simulink model "TEST_Datcom"  (R2020b)
settings: Solver=FixedStepAuto  StartTime=0.0  StopTime=100  FixedStep=DATCOM_DYN.Ts  RelTol=1e-3
undefined symbols (not defined in the file or in its folder): DATCOM_DYN, Earth, F, Light, MIL, statdyn, WGS84
libraries: aerolibadyn x3, aerolibwind2 x3, aerolibasang x3, aerolibactuator x3, shared6dof x2, aerolibatmos2 x2, aerolibconvert2 x2, pid_lib x1, simulink_extras x1, aerolibtransform2 x1
settings Model: Creator=sl  LastModifiedBy=sl
settings OptimizationCC: DefaultParameterBehavior=Inlined  EnhancedBackFolding=on  PassReuseOutputArgsAs=Individual arguments  ZeroExternalMemoryAtStartup=off  ZeroInternalMemoryAtStartup=off  OptimizeBlockOrder=speed  DifferentSizesBufferReuse=on  OptimizationCustomize=off  EfficientTunableParamExpr=on
settings DebuggingCC: ParameterTunabilityLossMsg=error
settings HardwareCC: ProdBitPerPointer=32  ProdBitPerSizeT=32  ProdBitPerPtrDiffT=32  ProdLargestAtomicInteger=Long  ProdWordSize=32  ProdHWDeviceType=ARM Compatible->ARM 10
settings SFSimCC: MATLABDynamicMemAlloc=off
settings RTWCC: Description=Embedded Coder  SystemTargetFile=ert.tlc  TemplateMakefile=ert_default_tmf
settings CodeAppCC: ForceParamTrailComments=on  IgnoreCustomStorageClasses=off  OperatorAnnotations=on  SimulinkDataObjDesc=on  SFDataObjDesc=on  InsertBlockDesc=on
settings ERTTargetCC: TargetLangStandard=C99 (ISO)  GenerateSampleERTMain=on  SupportContinuousTime=on  InlinedParameterPlacement=NonHierarchical  ERTCustomFileTemplate=example_file_process.tlc

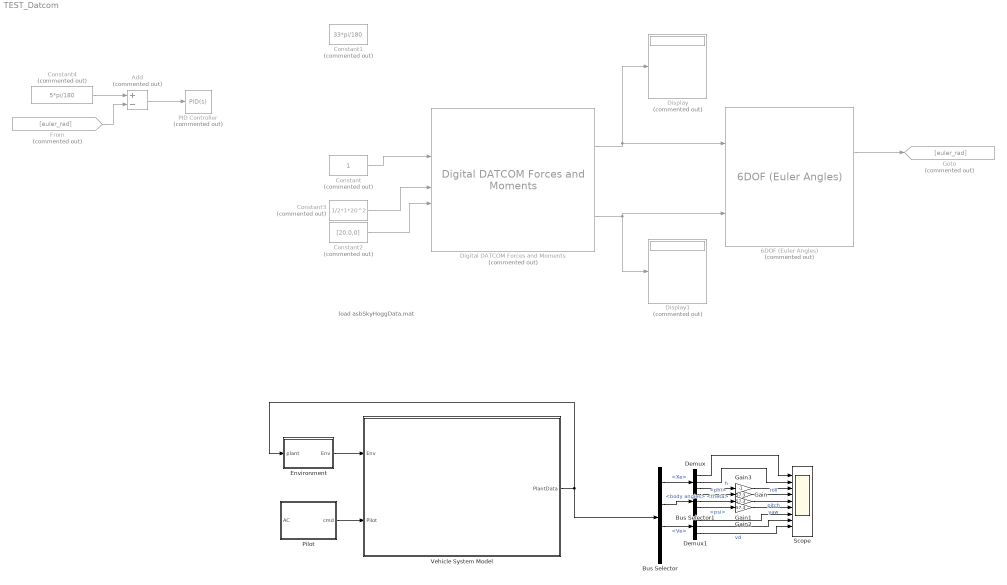
== system TEST_Datcom ==
  note: load asbSkyHoggData.mat
  6DOF (Euler Angles) : shared6dof/6DOF (Euler Angles)  Commented=on  units=Metric (MKS)  mtype=Fixed  rep=Euler Angles  xme_0=[0 0 0]  Vm_0=[0 0 0]  eul_0=[0 0 0]  pm_0=[0 0 0]  mass_0=1.0  mass_e=0.5  mass_f=2.0  inertia=eye(3)  inertia_e=eye(3)  inertia_f=2*eye(3)  k_quat=1.0  vre_flag=on  abi_flag=off  aMode=0  xme_statename=''  Vm_statename=''  eul_statename=''  quat_statename=''  pm_statename=''  mass_statename=''
      settings: SourceProductBaseCode=AE,PW,MT,UV,VE,VP
  Add : Sum  Commented=on  Inputs=+-
  Bus Selector : BusSelector  OutputSignals=Xe,body angles,Ve,Vb
  Bus Selector1 : BusSelector  OutputSignals=phi,theta,psi
  Constant : Constant  Commented=on
  Constant1 : Constant  Commented=on  Value=33*pi/180
  Constant2 : Constant  Commented=on  Value=[20,0,0]
  Constant3 : Constant  Commented=on  Value=1/2*1*20^2
  Constant4 : Constant  Commented=on  Value=5*pi/180
  Demux : Demux  Outputs=3
  Demux1 : Demux  Outputs=3
  Digital DATCOM Forces and Moments : aerolibadyn/Digital DATCOM Forces and Moments  Commented=on  units=Metric (MKS)  dcase=statdyn{1}  fmode=Body  buildno=0  imethod=Linear  emethod=None - clip  rmethod=Clip to Range  action=None
      settings: SourceProductBaseCode=AE
  Display : Display  Commented=on
  Display1 : Display  Commented=on
  Environment : Subsystem  TreatAsAtomicUnit=on
  From : From  Commented=on  GotoTag=euler_rad
  Gain : Gain  Gain=57.3
  Gain1 : Gain  Gain=57.3
  Gain2 : Gain  Gain=57.3
  Gain3 : Gain  Gain=-1
  Goto : Goto  Commented=on  GotoTag=euler_rad
  PID Controller : pid_lib/PID Controller  Commented=on  Controller=PID  Form=Parallel  TimeDomain=Continuous-time  UseExternalTs=off  SampleTime=-1  IntegratorMethod=Forward Euler  FilterMethod=Forward Euler  ControllerParametersSource=internal  P=1  I=1  D=0  UseFilter=on  N=100  TunerSelectOption=Transfer Function Based (PID Tuner App)  InitialConditionSource=internal  InitialConditionForIntegrator=0  InitialConditionForFilter=0  DifferentiatorICPrevScaledInput=0  ExternalReset=none  TrackingMode=off  Kt=1  LimitOutput=off  SatLimitsSource=internal  UpperSaturationLimit=inf  LowerSaturationLimit=-inf  LinearizeAsGain=on  AntiWindupMode=none  Kb=1  POutMin=[]  POutMax=[]  IOutMin=[]  IOutMax=[]  DOutMin=[]  DOutMax=[]  NOutMin=[]  NOutMax=[]  SumOutMin=[]  SumOutMax=[]  SaturationOutMin=[]  SaturationOutMax=[]  PParamMin=[]  PParamMax=[]  IParamMin=[]  IParamMax=[]  DParamMin=[]  DParamMax=[]  NParamMin=[]  NParamMax=[]  KbParamMin=[]  KbParamMax=[]  KtParamMin=[]  KtParamMax=[]  KbOutMin=[]  KbOutMax=[]  KtOutMin=[]  KtOutMax=[]  IntegratorOutMin=[]  IntegratorOutMax=[]  FilterOutMin=[]  FilterOutMax=[]  SumI1OutMin=[]  SumI1OutMax=[]  SumI2OutMin=[]  SumI2OutMax=[]  SumI3OutMin=[]  SumI3OutMax=[]  SumI4OutMin=[]  SumI4OutMax=[]  SumDOutMin=[]  SumDOutMax=[]  DifferentiatorOutMin=[]  DifferentiatorOutMax=[]  FilterDiffOutCoefMin=[]  FilterDiffOutCoefMax=[]  ReciprocalOutMin=[]  ReciprocalOutMax=[]  SumDenOutMin=[]  SumDenOutMax=[]  SumNumOutMin=[]  SumNumOutMax=[]  DivideOutMin=[]  DivideOutMax=[]  UdiffTsProdOutMin=[]  UdiffTsProdOutMax=[]  NTsProdOutMin=[]  NTsProdOutMax=[]  UintegralTsProdOutMin=[]  UintegralTsProdOutMax=[]  UngainTsProdOutMin=[]  UngainTsProdOutMax=[]  IntegratorContinuousStateAttributes=''  IntegratorStateMustResolveToSignalObject=off  IntegratorRTWStateStorageClass=Auto  FilterContinuousStateAttributes=''  FilterStateMustResolveToSignalObject=off  FilterRTWStateStorageClass=Auto  ParallelPVariant=InternalParameters  IdealPVariant=Disabled  IVariant=InternalParameters  DVariant=InternalParameters  IntegratorVariant=Continuous  SatVariant=Disabled  AWVariant=Passthrough  PCopyVariant=Disabled  TRVariant=Disabled  FdbkBlocksVariant=Forward  IdealPFdbkVariant=Disabled  SatFdbkVariant=Disabled  DerivativeFilterVariant=ContFilter  NVariant=InternalParameters  NCopyVariant=Disabled  FilterICVariant=InternalICsFilter  IntegratorICVariant=InternalICs  ExternalResetVariant=Disabled  TRSumVariant=Passthrough  SumFdbkVariant=Disabled  SumVariant=Sum_PID  TsampFilterVariant=InternalTs  TsampNgainVariant=Passthrough  TsampIntegralVariant=Passthrough  ExternalSaturationOutDataTypeStr=Inherit: Same as second input
  Pilot : Subsystem  TreatAsAtomicUnit=on
  Scope : Scope  NumInputPorts=9
  Vehicle System Model : Subsystem
      mask Display: image('asbSkyHogg.jpg',[.1 .1 .8 .8],'on')
  wires:
  ? -> Digital DATCOM Forces and Moments/1
  Digital DATCOM Forces and Moments/1 -> 6DOF (Euler Angles)/1, Display/1
  Digital DATCOM Forces and Moments/2 -> 6DOF (Euler Angles)/2, Display1/1
  Constant/1 -> Digital DATCOM Forces and Moments/3
  Constant2/1 -> Digital DATCOM Forces and Moments/6
  Constant3/1 -> Digital DATCOM Forces and Moments/5
  6DOF (Euler Angles)/3 -> Goto/1
  Constant4/1 -> Add/1
  From/1 -> Add/2
  Add/1 -> PID Controller/1
  Pilot/1(cmd) -> Vehicle System Model/2(Pilot)
  Environment/1(Env) -> Vehicle System Model/1(Env)
  Vehicle System Model/1(PlantData) -> Environment/1(plant), Bus Selector/1
  Bus Selector/1 -> Demux/1  "<Xe>"
  Bus Selector/2 -> Bus Selector1/1  "<body angles>"
  Bus Selector1/1 -> Gain/1  "<phi>"
  Bus Selector1/2 -> Gain1/1  "<theta>"
  Bus Selector1/3 -> Gain2/1  "<psi>"
  Demux/1 -> Scope/1
  Demux/2 -> Scope/2
  Demux/3 -> Gain3/1  "h"
  Gain/1 -> Scope/4  "roll"
  Gain1/1 -> Scope/5  "pitch"
  Gain2/1 -> Scope/6  "yaw"
  Gain3/1 -> Scope/3
  Bus Selector/3 -> Demux1/1  "<Ve>"
  Demux1/1 -> Scope/7
  Demux1/2 -> Scope/8
  Demux1/3 -> Scope/9  "vd"

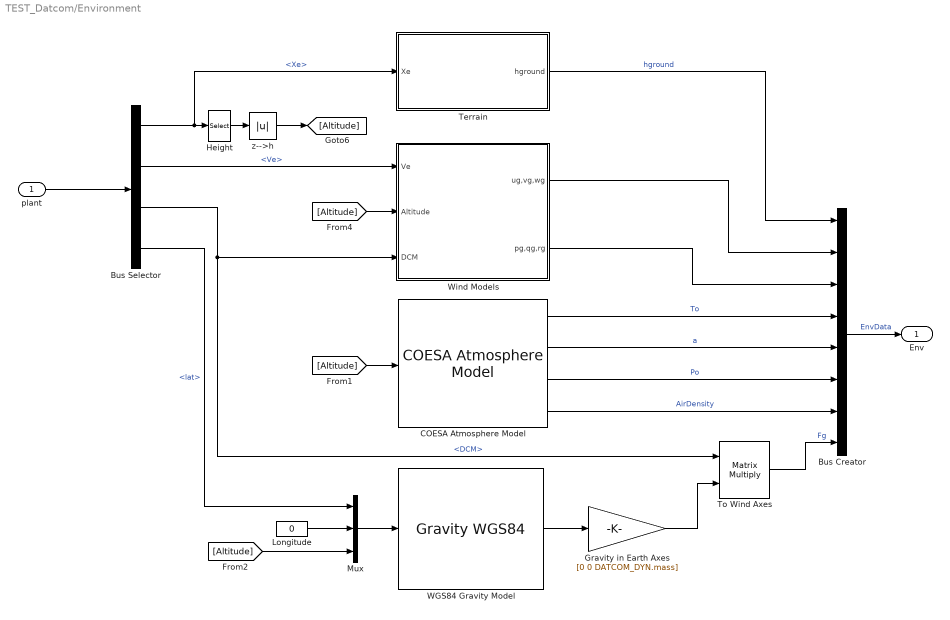
== system TEST_Datcom/Environment ==
  plant : Inport
  Bus Creator : BusCreator  Inputs='hground','WindVelocity','WindAngularRates','To','a','Po','AirDensity','Fg'
  Bus Selector : BusSelector  OutputSignals=Xe,Ve,DCM,lat
  COESA Atmosphere Model : aerolibatmos2/COESA Atmosphere Model  units=Metric (MKS)  spec=1976 COESA-extended U.S. Standard Atmosphere  model=Profile  profile_var=High temperature  profile_percent=1%  profile_alt=5 km (16404 ft)  envelope_var=High temperature  envelope_percent=1%  action=Warning
  Gravity in Earth Axes : Gain  Gain=[0 0 DATCOM_DYN.mass]  SaturateOnIntegerOverflow=on  OutDataTypeStr=Inherit: Same as input  ParamDataTypeStr=Inherit: Same as input
  Height : Selector  IndexMode=Zero-based  InputPortWidth=3  IndexOptions=Index vector (dialog)  Indices=2  OutputSizes=1
  Longitude : Constant  Value=0
  Mux : Mux  Inputs=3
  Terrain : Subsystem
  To Wind Axes : Product  Multiplication=Matrix(*)  InputSameDT=on  SaturateOnIntegerOverflow=on  OutDataTypeStr=Inherit: Same as first input
  "WGS84 Gravity Model  " : GravityWGS84
  Wind Models : Subsystem
  z-->h : Abs  SaturateOnIntegerOverflow=on
  Env : Outport  InitialOutput=0  VectorParamsAs1DForOutWhenUnconnected=off
  wires:
  Bus Selector/3 -> Wind Models/3(DCM), To Wind Axes/1  "<DCM>"
  Bus Selector/2 -> Wind Models/1(Ve)  "<Ve>"
  Bus Selector/1 -> Height/1, Terrain/1(Xe)  "<Xe>"
  [Altitude] -> COESA Atmosphere Model/1
  [Altitude] -> Mux/3
  [Altitude] -> Wind Models/2(Altitude)
  z-->h/1 -> [Altitude]
  plant/1 -> Bus Selector/1
  Bus Creator/1 -> Env/1  "EnvData"
  To Wind Axes/1 -> Bus Creator/8  "Fg"
  Gravity in Earth Axes/1 -> To Wind Axes/2
  "WGS84 Gravity Model  "/1 -> Gravity in Earth Axes/1
  Bus Selector/4 -> Mux/1  "<lat>"
  Height/1 -> z-->h/1
  COESA Atmosphere Model/1 -> Bus Creator/4  "To"
  COESA Atmosphere Model/3 -> Bus Creator/6  "Po"
  COESA Atmosphere Model/2 -> Bus Creator/5  "a"
  COESA Atmosphere Model/4 -> Bus Creator/7  "AirDensity"
  Wind Models/2(pg,qg,rg) -> Bus Creator/3
  Wind Models/1(ug,vg,wg) -> Bus Creator/2
  Terrain/1(hground) -> Bus Creator/1  "hground"
  Mux/1 -> "WGS84 Gravity Model  "/1
  Longitude/1 -> Mux/2

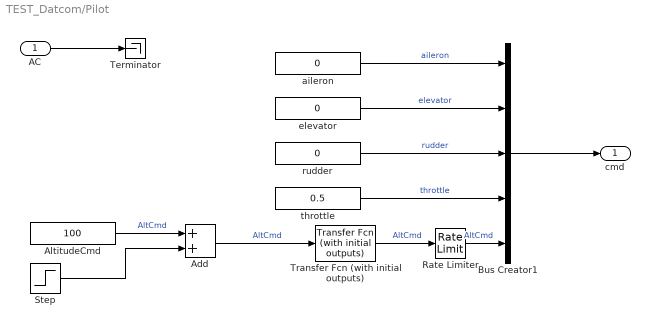
== system TEST_Datcom/Pilot ==
  AC : Inport
  Add : Sum
  AltitudeCmd : Constant  Value=100  OutDataTypeStr=double
  Bus Creator1 : BusCreator  Inputs=5
  Rate Limiter : RateLimiter  RisingSlewLimit=500/3/60  SampleTimeMode=inherited  InitialCondition=2000
  Step : Step  Time=5  After=50  SampleTime=0
  Terminator : Terminator
  Transfer Fcn (with initial outputs) : simulink_extras/Additional Linear/Transfer Fcn (with initial outputs)  N=.25  D=[1,.25]  Y0=2000  U0=2000
      settings: SourceProductName=Simulink Extras
  aileron : Constant  Value=0  OutDataTypeStr=single
  elevator : Constant  Value=0  OutDataTypeStr=single
  rudder : Constant  Value=0  OutDataTypeStr=single
  throttle : Constant  Value=0.5  OutDataTypeStr=double
  cmd : Outport  VectorParamsAs1DForOutWhenUnconnected=off
  wires:
  elevator/1 -> Bus Creator1/2  "elevator"
  aileron/1 -> Bus Creator1/1  "aileron"
  throttle/1 -> Bus Creator1/4  "throttle"
  rudder/1 -> Bus Creator1/3  "rudder"
  Bus Creator1/1 -> cmd/1
  AC/1 -> Terminator/1
  AltitudeCmd/1 -> Add/1  "AltCmd"
  Step/1 -> Add/2
  Add/1 -> Transfer Fcn (with initial outputs)/1  "AltCmd"
  Rate Limiter/1 -> Bus Creator1/5  "AltCmd"
  Transfer Fcn (with initial outputs)/1 -> Rate Limiter/1  "AltCmd"

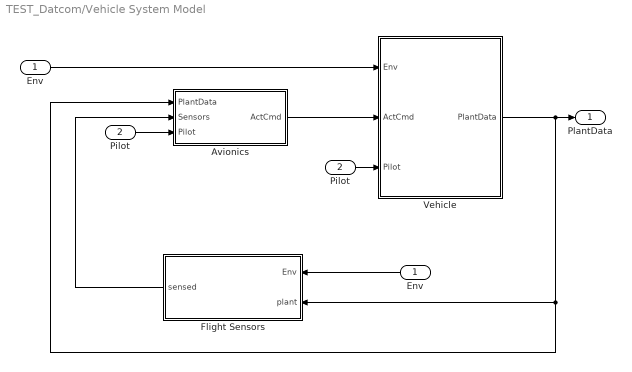
== system TEST_Datcom/Vehicle System Model ==
  Env : Inport
  Pilot : Inport  Port=2
  Avionics : Subsystem
  "Env " : InportShadow
  Flight Sensors : Subsystem
  "Pilot " : InportShadow  Port=2
  Vehicle : Subsystem
  PlantData : Outport  VectorParamsAs1DForOutWhenUnconnected=off
  wires:
  Env/1 -> Vehicle/1(Env)
  Vehicle/1(PlantData) -> Avionics/1(PlantData), Flight Sensors/2(plant), PlantData/1
  Flight Sensors/1(sensed) -> Avionics/2(Sensors)
  Avionics/1(ActCmd) -> Vehicle/2(ActCmd)
  Pilot/1 -> Vehicle/3(Pilot)
  "Env "/1 -> Flight Sensors/1(Env)
  "Pilot "/1 -> Avionics/3(Pilot)

== system TEST_Datcom/Environment/Terrain ==
  note: This part of the system defines the interface for the terrain model that will be developed in detail later on.
  Xe : Inport
  Terminator : Terminator
  hground_value : Constant  Value=0  OutDataTypeStr=single
  hground : Outport  Unit=m  VectorParamsAs1DForOutWhenUnconnected=off
  wires:
  hground_value/1 -> hground/1  "hground"
  Xe/1 -> Terminator/1

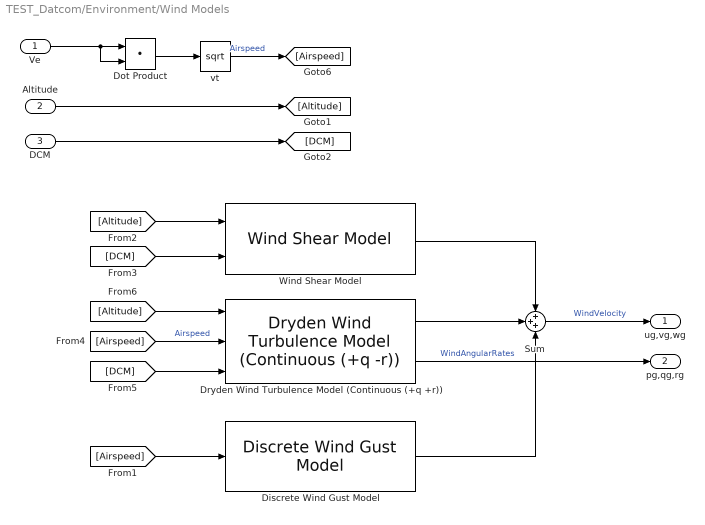
== system TEST_Datcom/Environment/Wind Models ==
  Ve : Inport
  Altitude : Inport  Port=2
  DCM : Inport  Port=3
  Discrete Wind Gust Model : aerolibwind2/Discrete Wind Gust Model  units=Metric (MKS)  Gx=off  Gy=off  Gz=off  t_0=20  d_m=[120 120 80]  v_m=[3.5 3.0 3.0]
      settings: SourceProductName=Aerospace Blockset
  Dot Product : DotProduct  OutDataTypeStr=Inherit: Inherit via internal rule
  Dryden Wind Turbulence Model (Continuous (+q +r)) : aerolibwind2/Dryden Wind Turbulence Model  (Continuous (+q -r))  units=Metric (MKS)  spec=MIL-F-8785C  model=Continuous Dryden (+q +r)  W20=5  Wdeg=0  TurbProb=10^-2 - Light  L_high=533.4  Wingspan=4  ts=DATCOM_DYN.Ts  Seed=[23341 23342 23343 23344]  T_on=off
      settings: SourceProductName=Aerospace Blockset
  Sum : Sum  Inputs=+++  InputSameDT=on  SaturateOnIntegerOverflow=on  OutDataTypeStr=Inherit: Same as first input
  Wind Shear Model : aerolibwind2/Wind Shear Model  units=Metric (MKS)  phase=Category C - Terminal Flight Phase  W_20=1  Wdeg=0
      settings: SourceProductName=Aerospace Blockset
  vt : Sqrt  SaturateOnIntegerOverflow=on
  ug,vg,wg : Outport  Unit=m/s  VectorParamsAs1DForOutWhenUnconnected=off
  pg,qg,rg : Outport  Port=2  Unit=rad/second  VectorParamsAs1DForOutWhenUnconnected=off
  wires:
  [Altitude] -> Dryden Wind Turbulence Model (Continuous (+q +r))/1
  [DCM] -> Dryden Wind Turbulence Model (Continuous (+q +r))/3
  [DCM] -> Wind Shear Model/2
  DCM/1 -> [DCM]
  [Altitude] -> Wind Shear Model/1
  Altitude/1 -> [Altitude]
  [Airspeed] -> Discrete Wind Gust Model/1
  vt/1 -> [Airspeed]  "Airspeed"
  Dot Product/1 -> vt/1
  Dryden Wind Turbulence Model (Continuous (+q +r))/2 -> pg,qg,rg/1  "WindAngularRates"
  [Airspeed] -> Dryden Wind Turbulence Model (Continuous (+q +r))/2  "Airspeed"
  Sum/1 -> ug,vg,wg/1  "WindVelocity"
  Discrete Wind Gust Model/1 -> Sum/3
  Dryden Wind Turbulence Model (Continuous (+q +r))/1 -> Sum/2
  Wind Shear Model/1 -> Sum/1
  Ve/1 -> Dot Product/2, Dot Product/1

== system TEST_Datcom/Vehicle System Model/Avionics ==
  PlantData : Inport
  Sensors : Inport  Port=2
  Pilot : Inport  Port=3
  Autopilot : Subsystem
  ActCmd : Outport  VectorParamsAs1DForOutWhenUnconnected=off
  wires:
  Autopilot/1(cmd) -> ActCmd/1

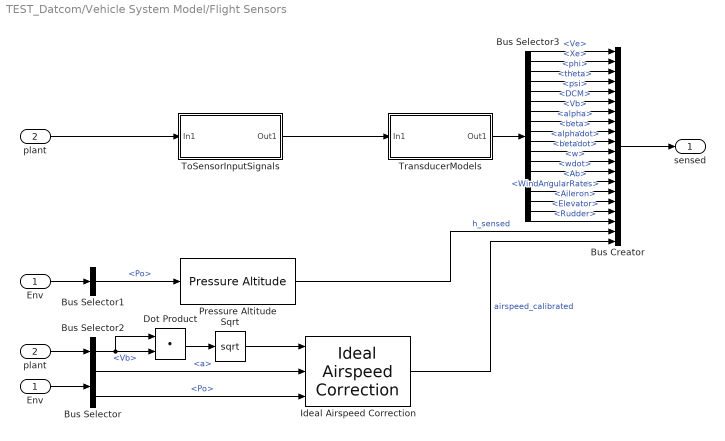
== system TEST_Datcom/Vehicle System Model/Flight Sensors ==
  Env : Inport
  plant : Inport  Port=2
  Bus Creator : BusCreator  Inputs=20
  Bus Selector : BusSelector  OutputSignals=a,Po
  Bus Selector1 : BusSelector  OutputSignals=Po
  Bus Selector2 : BusSelector  OutputSignals=Vb
  Bus Selector3 : BusSelector  OutputSignals=Ve,Xe,body angles.phi,body angles.theta,body angles.psi,DCM,Vb,alpha,beta,alphadot,betadot,w,wdot,Ab,WindAngularRates,Act_positions.Aileron,Act_positions.Elevator,Act_positions.Rudder
  Dot Product : DotProduct  InputSameDT=on  OutDataTypeStr=Inherit: Inherit via internal rule
  "Env " : InportShadow
  Ideal Airspeed Correction : aerolibasang/Ideal Airspeed Correction  units=Metric (MKS)  vel_in=TAS  vel_out_tas=CAS  vel_out_eas=CAS  vel_out_cas=TAS  method=Table Lookup  SubOnly=off  action=Error
      settings: SourceProductName=Aerospace Blockset
  Pressure Altitude : aerolibatmos2/Pressure Altitude  units=Metric (MKS)  action=Warning
      settings: SourceProductName=Aerospace Blockset
  Sqrt : Sqrt  SaturateOnIntegerOverflow=on
  ToSensorInputSignals : Subsystem
  TransducerModels : Subsystem
  "plant " : InportShadow  Port=2
  sensed : Outport  VectorParamsAs1DForOutWhenUnconnected=off
  wires:
  ToSensorInputSignals/1(Out1) -> TransducerModels/1(In1)
  Env/1 -> Bus Selector/1
  TransducerModels/1(Out1) -> Bus Selector3/1
  plant/1 -> ToSensorInputSignals/1(In1)
  Bus Selector/1 -> Ideal Airspeed Correction/2  "<a>"
  Bus Selector/2 -> Ideal Airspeed Correction/3  "<Po>"
  Bus Selector1/1 -> Pressure Altitude/1  "<Po>"
  "Env "/1 -> Bus Selector1/1
  "plant "/1 -> Bus Selector2/1
  Dot Product/1 -> Sqrt/1
  Sqrt/1 -> Ideal Airspeed Correction/1
  Bus Selector2/1 -> Dot Product/2, Dot Product/1  "<Vb>"
  Bus Selector3/1 -> Bus Creator/1  "<Ve>"
  Bus Selector3/2 -> Bus Creator/2  "<Xe>"
  Bus Selector3/3 -> Bus Creator/3  "<phi>"
  Bus Selector3/4 -> Bus Creator/4  "<theta>"
  Bus Selector3/5 -> Bus Creator/5  "<psi>"
  Bus Selector3/6 -> Bus Creator/6  "<DCM>"
  Bus Selector3/7 -> Bus Creator/7  "<Vb>"
  Bus Selector3/8 -> Bus Creator/8  "<alpha>"
  Bus Selector3/9 -> Bus Creator/9  "<beta>"
  Bus Selector3/10 -> Bus Creator/10  "<alphadot>"
  Bus Selector3/11 -> Bus Creator/11  "<betadot>"
  Bus Selector3/12 -> Bus Creator/12  "<w>"
  Bus Selector3/13 -> Bus Creator/13  "<wdot>"
  Bus Selector3/14 -> Bus Creator/14  "<Ab>"
  Bus Creator/1 -> sensed/1
  Bus Selector3/15 -> Bus Creator/15  "<WindAngularRates>"
  Bus Selector3/16 -> Bus Creator/16  "<Aileron>"
  Bus Selector3/17 -> Bus Creator/17  "<Elevator>"
  Bus Selector3/18 -> Bus Creator/18  "<Rudder>"
  Pressure Altitude/1 -> Bus Creator/19  "h_sensed"
  Ideal Airspeed Correction/1 -> Bus Creator/20  "airspeed_calibrated"

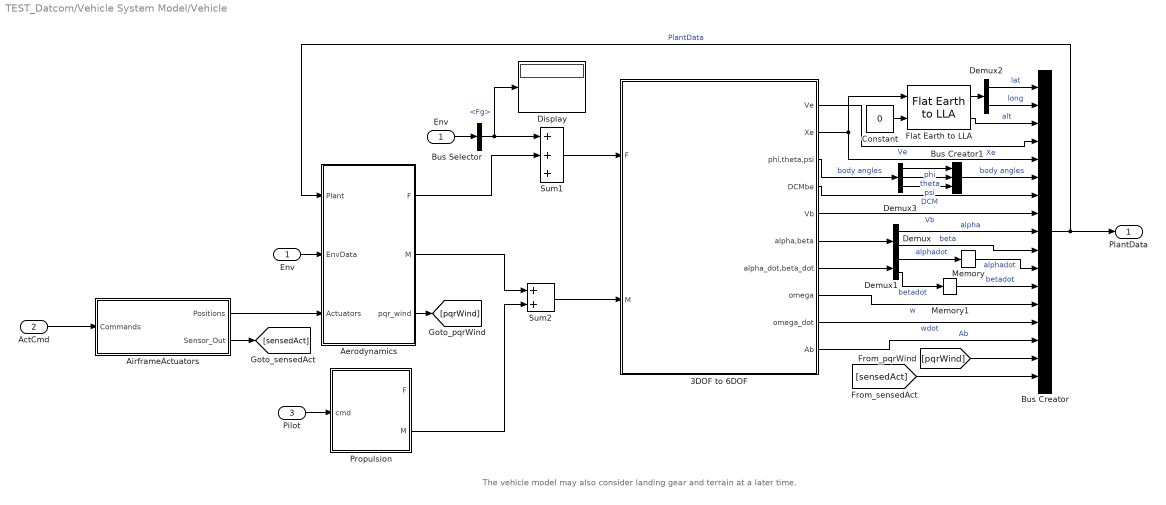
== system TEST_Datcom/Vehicle System Model/Vehicle ==
  note: The vehicle model may also consider landing gear and terrain at a later time.
  Env : Inport
  ActCmd : Inport  Port=2
  Pilot : Inport  Port=3
  3DOF to 6DOF : Subsystem
  Aerodynamics : Subsystem
  AirframeActuators : Subsystem
  Bus Creator : BusCreator  Inputs=17
  Bus Creator1 : BusCreator  Inputs=3
  Bus Selector : BusSelector  OutputSignals=Fg
  Constant : Constant  Value=0
  Demux : Demux  Outputs=2
  Demux1 : Demux  Outputs=2
  Demux2 : Demux  Outputs=2
  Demux3 : Demux  Outputs=3
  Display : Display
  "Env " : InportShadow
  Flat Earth to LLA : aerolibtransform2/Flat Earth to LLA  units=Metric (MKS)  ptype=Earth (WGS84)  F=1/298.257223563  R=6378137  refPosPort=off  LL0=DATCOM_DYN.LatLong0  psi=DATCOM_DYN.heading0
  Memory : Memory  LinearizeMemory=on
  Memory1 : Memory  LinearizeMemory=on
  Propulsion : Subsystem
      settings: RTWSystemCode=Inline
  Sum1 : Sum  Inputs=+++  InputSameDT=on  SaturateOnIntegerOverflow=on  OutDataTypeStr=Inherit: Same as first input
  Sum2 : Sum  InputSameDT=on  SaturateOnIntegerOverflow=on  OutDataTypeStr=Inherit: Same as first input
  PlantData : Outport  VectorParamsAs1DForOutWhenUnconnected=off
  wires:
  Sum1/1 -> 3DOF to 6DOF/1(F)
  Sum2/1 -> 3DOF to 6DOF/2(M)
  3DOF to 6DOF/3(phi,theta,psi) -> Demux3/1  "body angles"
  3DOF to 6DOF/4(DCMbe) -> Bus Creator/7  "DCM"
  3DOF to 6DOF/5(Vb) -> Bus Creator/8  "Vb"
  3DOF to 6DOF/6(alpha,beta) -> Demux/1
  3DOF to 6DOF/7(alpha_dot,beta_dot) -> Demux1/1
  3DOF to 6DOF/9(omega_dot) -> Bus Creator/14  "wdot"
  3DOF to 6DOF/10(Ab) -> Bus Creator/15  "Ab"
  Bus Creator/1 -> Aerodynamics/1(Plant), PlantData/1  "PlantData"
  Aerodynamics/1(F) -> Sum1/2
  Aerodynamics/2(M) -> Sum2/1
  Bus Selector/1 -> Display/1, Sum1/1  "<Fg>"
  Env/1 -> Aerodynamics/2(EnvData)
  ActCmd/1 -> AirframeActuators/1(Commands)
  Pilot/1 -> Propulsion/1(cmd)
  "Env "/1 -> Bus Selector/1
  AirframeActuators/1(Positions) -> Aerodynamics/3(Actuators)
  Aerodynamics/3(pqr_wind) -> [pqrWind]
  [pqrWind] -> Bus Creator/16
  AirframeActuators/2(Sensor_Out) -> [sensedAct]
  [sensedAct] -> Bus Creator/17
  Constant/1 -> Flat Earth to LLA/2
  Flat Earth to LLA/2 -> Bus Creator/3  "alt"
  Flat Earth to LLA/1 -> Demux2/1
  Demux2/1 -> Bus Creator/1  "lat"
  Demux2/2 -> Bus Creator/2  "long"
  Demux1/1 -> Memory/1  "alphadot"
  Demux1/2 -> Memory1/1  "betadot"
  Demux3/1 -> Bus Creator1/1  "phi"
  Demux3/2 -> Bus Creator1/2  "theta"
  Demux3/3 -> Bus Creator1/3  "psi"
  Bus Creator1/1 -> Bus Creator/6  "body angles"
  3DOF to 6DOF/8(omega) -> Bus Creator/13  "w"
  Demux/2 -> Bus Creator/10  "beta"
  Demux/1 -> Bus Creator/9  "alpha"
  Memory/1 -> Bus Creator/11  "alphadot"
  Memory1/1 -> Bus Creator/12  "betadot"
  3DOF to 6DOF/1(Ve) -> Bus Creator/4  "Ve"
  3DOF to 6DOF/2(Xe) -> Flat Earth to LLA/1, Bus Creator/5  "Xe"
  Propulsion/2(M) -> Sum2/2

== system TEST_Datcom/Vehicle System Model/Avionics/Autopilot ==
  Bus Creator1 : BusCreator  Inputs=3
  Ground : Ground
  Ground2 : Ground
  cmd : Outport  VectorParamsAs1DForOutWhenUnconnected=off
  wires:
  Bus Creator1/1 -> cmd/1
  Ground2/1 -> Bus Creator1/3  "Rudder"
  Ground/1 -> Bus Creator1/1  "Aileron"
  ? -> Bus Creator1/2  "Elevator"

== system TEST_Datcom/Vehicle System Model/Flight Sensors/ToSensorInputSignals ==
  note: This part of the system defines the interface for the measurement noise model that
      |  will be developed in detail later on.
  In1 : Inport
  Out1 : Outport  VectorParamsAs1DForOutWhenUnconnected=off
  wires:
  In1/1 -> Out1/1

== system TEST_Datcom/Vehicle System Model/Flight Sensors/TransducerModels ==
  note: This part of the system defines the interface for the transducers model that
      |  will be developed in detail later on.
  In1 : Inport
  Out1 : Outport  VectorParamsAs1DForOutWhenUnconnected=off
  wires:
  In1/1 -> Out1/1

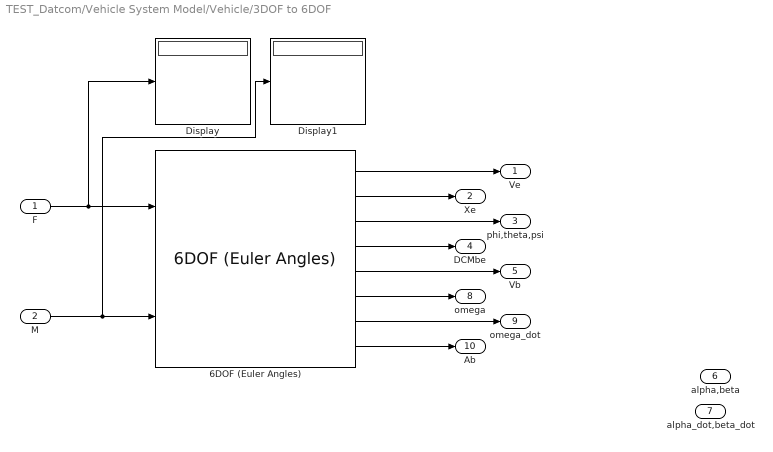
== system TEST_Datcom/Vehicle System Model/Vehicle/3DOF to 6DOF ==
  F : Inport
  M : Inport  Port=2
  6DOF (Euler Angles) : shared6dof/6DOF (Euler Angles)  units=Metric (MKS)  mtype=Fixed  rep=Euler Angles  xme_0=[0 0 0]  Vm_0=[30 0 0]  eul_0=[0 0 0]  pm_0=[0 0 0]  mass_0=DATCOM_DYN.mass  mass_e=0.5  mass_f=2.0  inertia=DATCOM_DYN.inertia  inertia_e=eye(3)  inertia_f=2*eye(3)  k_quat=1.0  vre_flag=on  abi_flag=off  aMode=0  xme_statename=''  Vm_statename=''  eul_statename=''  quat_statename=''  pm_statename=''  mass_statename=''
      settings: SourceProductBaseCode=AE,PW,MT,UV,VE,VP
  Display : Display
  Display1 : Display
  Ve : Outport  Unit=m/s  VectorParamsAs1DForOutWhenUnconnected=off
  Xe : Outport  Port=2  Unit=m  VectorParamsAs1DForOutWhenUnconnected=off
  phi,theta,psi : Outport  Port=3  Unit=rad  VectorParamsAs1DForOutWhenUnconnected=off
  DCMbe : Outport  Port=4  VectorParamsAs1DForOutWhenUnconnected=off
  Vb : Outport  Port=5  Unit=m/s  VectorParamsAs1DForOutWhenUnconnected=off
  alpha,beta : Outport  Port=6  Unit=rad  VectorParamsAs1DForOutWhenUnconnected=off
  alpha_dot,beta_dot : Outport  Port=7  Unit=rad/s  VectorParamsAs1DForOutWhenUnconnected=off
  omega : Outport  Port=8  Unit=rad/s  VectorParamsAs1DForOutWhenUnconnected=off
  omega_dot : Outport  Port=9  Unit=rad/s^2  VectorParamsAs1DForOutWhenUnconnected=off
  Ab : Outport  Port=10  Unit=m/s^2  VectorParamsAs1DForOutWhenUnconnected=off
  wires:
  F/1 -> Display/1, 6DOF (Euler Angles)/1
  6DOF (Euler Angles)/6 -> omega/1
  6DOF (Euler Angles)/7 -> omega_dot/1
  6DOF (Euler Angles)/2 -> Xe/1
  6DOF (Euler Angles)/1 -> Ve/1
  ? -> alpha_dot,beta_dot/1
  6DOF (Euler Angles)/3 -> phi,theta,psi/1
  6DOF (Euler Angles)/5 -> Vb/1
  6DOF (Euler Angles)/8 -> Ab/1
  ? -> alpha,beta/1
  6DOF (Euler Angles)/4 -> DCMbe/1
  M/1 -> Display1/1, 6DOF (Euler Angles)/2

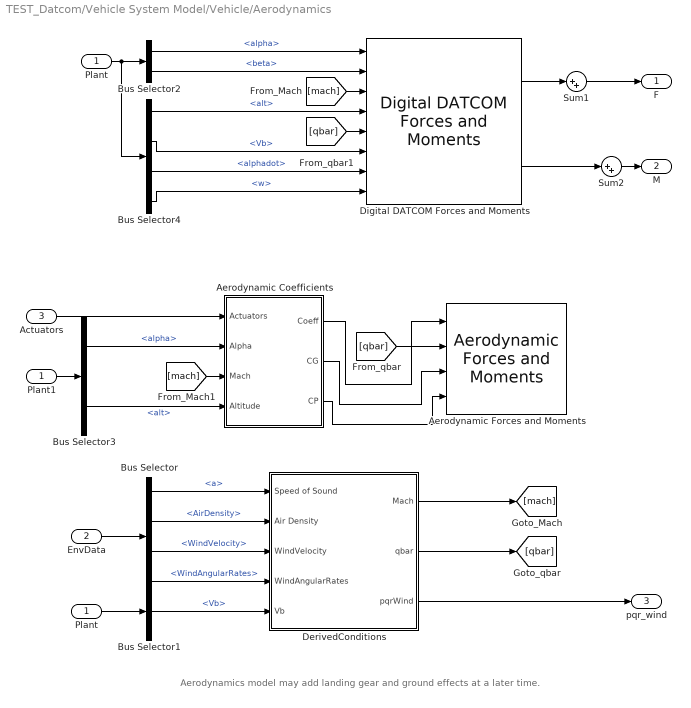
== system TEST_Datcom/Vehicle System Model/Vehicle/Aerodynamics ==
  note: Aerodynamics model may add landing gear and ground effects at a later time.
  Plant : Inport
  EnvData : Inport  Port=2
  Actuators : Inport  Port=3
  Aerodynamic Coefficients : Subsystem
  "Aerodynamic Forces and Moments " : aerolibadyn/Aerodynamic Forces and Moments   inputAxes=Body  outputForceAxes=Body  outputMomentAxes=Body  S=DATCOM_DYN.Sref  b=DATCOM_DYN.bref  cbar=DATCOM_DYN.cbar
      settings: SourceProductName=Aerospace Blockset
  Bus Selector : BusSelector  OutputSignals=a,AirDensity,WindVelocity,WindAngularRates
  Bus Selector1 : BusSelector  OutputSignals=Vb
  Bus Selector2 : BusSelector  OutputSignals=alpha,beta
  Bus Selector3 : BusSelector  OutputSignals=alpha,alt
  Bus Selector4 : BusSelector  OutputSignals=alt,Vb,alphadot,w
  DerivedConditions : Subsystem
  Digital DATCOM Forces and Moments : aerolibadyn/Digital DATCOM Forces and Moments  units=Metric (MKS)  dcase=statdyn{1}  fmode=Body  buildno=0  imethod=Linear  emethod=Linear  rmethod=Linear Extrapolation  action=None
      settings: SourceProductName=Aerospace Blockset
  "Plant " : InportShadow
  Plant1 : InportShadow
  Sum1 : Sum  Inputs=|++
  Sum2 : Sum  Inputs=|++
  F : Outport  Unit=N  VectorParamsAs1DForOutWhenUnconnected=off
  M : Outport  Port=2  Unit=N*m  VectorParamsAs1DForOutWhenUnconnected=off
  pqr_wind : Outport  Port=3  Unit=rad/s  VectorParamsAs1DForOutWhenUnconnected=off
  wires:
  Digital DATCOM Forces and Moments/1 -> Sum1/1
  Digital DATCOM Forces and Moments/2 -> Sum2/1
  Aerodynamic Coefficients/1(Coeff) -> "Aerodynamic Forces and Moments "/1
  Sum1/1 -> F/1
  Sum2/1 -> M/1
  EnvData/1 -> Bus Selector/1
  Bus Selector/1 -> DerivedConditions/1(Speed of Sound)  "<a>"
  Bus Selector/2 -> DerivedConditions/2(Air Density)  "<AirDensity>"
  Bus Selector/3 -> DerivedConditions/3(WindVelocity)  "<WindVelocity>"
  Bus Selector/4 -> DerivedConditions/4(WindAngularRates)  "<WindAngularRates>"
  "Plant "/1 -> Bus Selector1/1
  Bus Selector1/1 -> DerivedConditions/5(Vb)  "<Vb>"
  Plant/1 -> Bus Selector2/1, Bus Selector4/1
  Bus Selector2/1 -> Digital DATCOM Forces and Moments/1  "<alpha>"
  Bus Selector2/2 -> Digital DATCOM Forces and Moments/2  "<beta>"
  Plant1/1 -> Bus Selector3/1
  Bus Selector3/1 -> Aerodynamic Coefficients/2(Alpha)  "<alpha>"
  DerivedConditions/1(Mach) -> [mach]
  [mach] -> Digital DATCOM Forces and Moments/3
  Aerodynamic Coefficients/2(CG) -> "Aerodynamic Forces and Moments "/3
  Aerodynamic Coefficients/3(CP) -> "Aerodynamic Forces and Moments "/4
  DerivedConditions/2(qbar) -> [qbar]
  [qbar] -> "Aerodynamic Forces and Moments "/2
  [qbar] -> Digital DATCOM Forces and Moments/5
  Bus Selector4/2 -> Digital DATCOM Forces and Moments/6  "<Vb>"
  Bus Selector4/1 -> Digital DATCOM Forces and Moments/4  "<alt>"
  DerivedConditions/3("pqrWind ") -> pqr_wind/1
  Bus Selector4/3 -> Digital DATCOM Forces and Moments/7  "<alphadot>"
  Bus Selector4/4 -> Digital DATCOM Forces and Moments/8  "<w>"
  Actuators/1 -> Aerodynamic Coefficients/1(Actuators)
  Bus Selector3/2 -> Aerodynamic Coefficients/4(Altitude)  "<alt>"
  [mach] -> Aerodynamic Coefficients/3(Mach)

== system TEST_Datcom/Vehicle System Model/Vehicle/AirframeActuators ==
  Commands : Inport
  Bus Creator : BusCreator  Inputs=3
  Bus Selector1 : BusSelector  OutputSignals=Aileron,Elevator,Rudder
  Nonlinear Second-Order Actuator : aerolibactuator/Nonlinear Second-Order Actuator  wn_fin=DATCOM_DYN.wn_act  z_fin=DATCOM_DYN.z_act  fin_max=DATCOM_DYN.maxdef_aileron  fin_min=DATCOM_DYN.mindef_aileron  fin_maxrate=Inf  fin_act_0=0  fin_act_vel=0
      settings: SourceProductName=Aerospace Blockset
  Nonlinear Second-Order Actuator1 : aerolibactuator/Nonlinear Second-Order Actuator  wn_fin=DATCOM_DYN.wn_act  z_fin=DATCOM_DYN.z_act  fin_max=DATCOM_DYN.maxdef_elevator  fin_min=DATCOM_DYN.mindef_elevator  fin_maxrate=Inf  fin_act_0=0  fin_act_vel=0
      settings: SourceProductName=Aerospace Blockset
  Nonlinear Second-Order Actuator2 : aerolibactuator/Nonlinear Second-Order Actuator  wn_fin=DATCOM_DYN.wn_act  z_fin=DATCOM_DYN.z_act  fin_max=DATCOM_DYN.maxdef_rudder  fin_min=DATCOM_DYN.mindef_rudder  fin_maxrate=Inf  fin_act_0=0  fin_act_vel=0
      settings: SourceProductName=Aerospace Blockset
  Positions : Outport  VectorParamsAs1DForOutWhenUnconnected=off
  Sensor_Out : Outport  Port=2  VectorParamsAs1DForOutWhenUnconnected=off
  wires:
  Commands/1 -> Bus Selector1/1
  Bus Selector1/1 -> Nonlinear Second-Order Actuator/1  "<Aileron>"
  Bus Selector1/2 -> Nonlinear Second-Order Actuator1/1  "<Elevator>"
  Bus Selector1/3 -> Nonlinear Second-Order Actuator2/1  "<Rudder>"
  Nonlinear Second-Order Actuator2/1 -> Bus Creator/3  "Rudder"
  Bus Creator/1 -> Sensor_Out/1, Positions/1  "Act_positions"
  Nonlinear Second-Order Actuator/1 -> Bus Creator/1  "Aileron"
  Nonlinear Second-Order Actuator1/1 -> Bus Creator/2  "Elevator"

== system TEST_Datcom/Vehicle System Model/Vehicle/Propulsion ==
  cmd : Inport  SampleTime=DATCOM_DYN.Ts
  Bus Selector2 : BusSelector  OutputSignals=throttle
  Mux : Mux  Inputs=[1 2]
  ThrustX : Lookup_n-D  NumberOfTableDimensions=1  LookupTableObject=''  BreakpointsForDimension1=(1/6)*(3+([-3:3]))  IndexSearchMethod=Linear search  BeginIndexSearchUsingPreviousIndexResult=on  Table=DATCOM_DYN.Thrust*(1+tanh([-3:3]))  ExtrapMethod=Clip  InputSameDT=on
  Thrust_LMN : Constant  Value=[0, 0, 0]  SampleTime=DATCOM_DYN.Ts
  Thrust_YZ : Constant  Value=[0, 0]  SampleTime=DATCOM_DYN.Ts
  F : Outport  Unit=N  VectorParamsAs1DForOutWhenUnconnected=off
  M : Outport  Port=2  Unit=N*m  VectorParamsAs1DForOutWhenUnconnected=off
  wires:
  ThrustX/1 -> Mux/1
  Thrust_YZ/1 -> Mux/2
  Mux/1 -> F/1
  cmd/1 -> Bus Selector2/1
  Thrust_LMN/1 -> M/1
  Bus Selector2/1 -> ThrustX/1  "<throttle>"

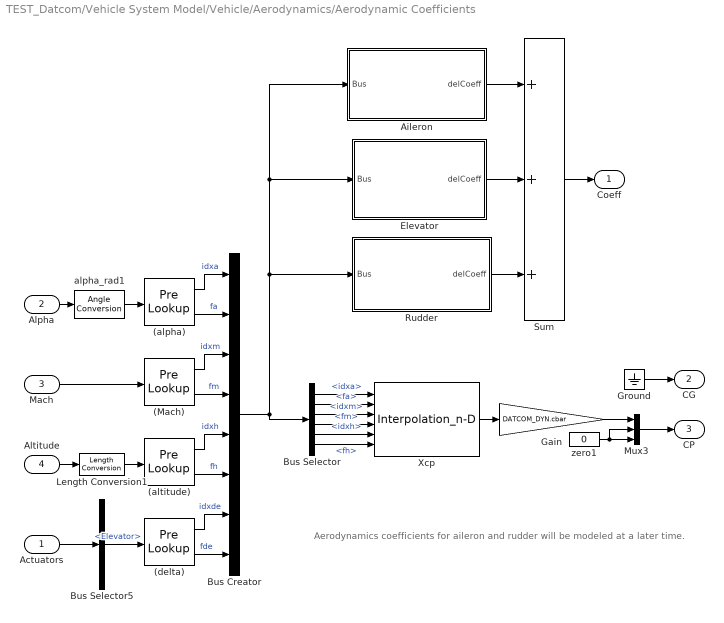
== system TEST_Datcom/Vehicle System Model/Vehicle/Aerodynamics/Aerodynamic Coefficients ==
  note: Aerodynamics coefficients for aileron and rudder will be modeled at a later time.
  Actuators : Inport
  Alpha : Inport  Port=2
  Mach : Inport  Port=3
  Altitude : Inport  Port=4
  (Mach) : PreLookup  BreakpointsData=statdyn{1}.mach  BeginIndexSearchUsingPreviousIndexResult=on  ExtrapMethod=Linear  IndexDataTypeStr=int32  FractionDataTypeStr=double
  (alpha) : PreLookup  BreakpointsData=statdyn{1}.alpha  BeginIndexSearchUsingPreviousIndexResult=on  ExtrapMethod=Linear  IndexDataTypeStr=int32  FractionDataTypeStr=double
  (altitude) : PreLookup  BreakpointsData=statdyn{1}.alt  BeginIndexSearchUsingPreviousIndexResult=on  ExtrapMethod=Linear  IndexDataTypeStr=int32  FractionDataTypeStr=double
  (delta) : PreLookup  BreakpointsData=statdyn{1}.delta  BeginIndexSearchUsingPreviousIndexResult=on  ExtrapMethod=Linear  IndexDataTypeStr=int32  FractionDataTypeStr=double
  Aileron : Subsystem
  Bus Creator : BusCreator  Inputs=8
  Bus Selector : BusSelector  OutputSignals=idxa,fa,idxm,fm,idxh,fh
  Bus Selector5 : BusSelector  OutputSignals=Elevator
  Elevator : Subsystem
  Gain : Gain  Gain=DATCOM_DYN.cbar
  Ground : Ground
  Length Conversion1 : aerolibconvert2/Length Conversion  IU=m  OU=ft
  Mux3 : Mux  Inputs=3
  Rudder : Subsystem
  Sum : Sum  Inputs=3  InputSameDT=on  SaturateOnIntegerOverflow=on  OutDataTypeStr=Inherit: Same as first input
  Xcp : Interpolation_n-D  NumberOfTableDimensions=3  Table="permute(statdyn{1}.xcp,[1  2  3])"  OutDataTypeStr=double
      settings: InputPortMap=u0,u1,u2,u3,u4,u5
  alpha_rad1 : aerolibconvert2/Angle Conversion  IU=rad  OU=deg
  zero1 : Constant  Value=0
  Coeff : Outport  InitialOutput=0  VectorParamsAs1DForOutWhenUnconnected=off
  CG : Outport  Port=2  PortDimensions=3  InitialOutput=0  VectorParamsAs1DForOutWhenUnconnected=off
  CP : Outport  Port=3  PortDimensions=3  InitialOutput=0  VectorParamsAs1DForOutWhenUnconnected=off
  wires:
  Sum/1 -> Coeff/1
  Actuators/1 -> Bus Selector5/1
  Ground/1 -> CG/1
  Mux3/1 -> CP/1
  Xcp/1 -> Gain/1
  zero1/1 -> Mux3/2, Mux3/3
  Gain/1 -> Mux3/1
  (alpha)/2 -> Bus Creator/2  "fa"
  (Mach)/2 -> Bus Creator/4  "fm"
  (altitude)/2 -> Bus Creator/6  "fh"
  (altitude)/1 -> Bus Creator/5  "idxh"
  (Mach)/1 -> Bus Creator/3  "idxm"
  (alpha)/1 -> Bus Creator/1  "idxa"
  Bus Selector/1 -> Xcp/1  "<idxa>"
  Bus Selector/2 -> Xcp/2  "<fa>"
  Bus Selector/3 -> Xcp/3  "<idxm>"
  Bus Selector/4 -> Xcp/4  "<fm>"
  Bus Selector/5 -> Xcp/5  "<idxh>"
  Bus Selector/6 -> Xcp/6  "<fh>"
  Bus Creator/1 -> Bus Selector/1, Elevator/1(Bus), Aileron/1(Bus), Rudder/1(Bus)
  Mach/1 -> (Mach)/1
  Altitude/1 -> Length Conversion1/1
  Length Conversion1/1 -> (altitude)/1
  Alpha/1 -> alpha_rad1/1
  alpha_rad1/1 -> (alpha)/1
  Aileron/1(delCoeff) -> Sum/1
  Elevator/1(delCoeff) -> Sum/2
  Rudder/1(delCoeff) -> Sum/3
  (delta)/1 -> Bus Creator/7  "idxde"
  (delta)/2 -> Bus Creator/8  "fde"
  Bus Selector5/1 -> (delta)/1  "<Elevator>"

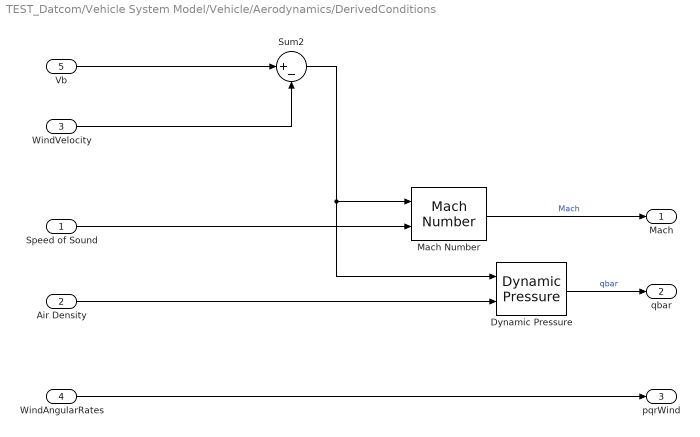
== system TEST_Datcom/Vehicle System Model/Vehicle/Aerodynamics/DerivedConditions ==
  Speed of Sound : Inport
  Air Density : Inport  Port=2
  WindVelocity : Inport  Port=3  PortDimensions=3
  WindAngularRates : Inport  Port=4  PortDimensions=3
  Vb : Inport  Port=5  PortDimensions=3
  Dynamic Pressure : aerolibasang/Dynamic Pressure
  Mach Number : aerolibasang/Mach Number
      settings: SourceProductName=Aerospace Blockset
  Sum2 : Sum  Inputs=|+-  InputSameDT=on  SaturateOnIntegerOverflow=on  OutDataTypeStr=Inherit: Same as first input
  Mach : Outport  VectorParamsAs1DForOutWhenUnconnected=off
  qbar : Outport  Port=2  InitialOutput=0  VectorParamsAs1DForOutWhenUnconnected=off
  "pqrWind " : Outport  Port=3  VectorParamsAs1DForOutWhenUnconnected=off
  wires:
  Speed of Sound/1 -> Mach Number/2
  Mach Number/1 -> Mach/1  "Mach"
  Air Density/1 -> Dynamic Pressure/2
  Dynamic Pressure/1 -> qbar/1  "qbar"
  WindAngularRates/1 -> "pqrWind "/1
  Vb/1 -> Sum2/1
  Sum2/1 -> Dynamic Pressure/1, Mach Number/1
  WindVelocity/1 -> Sum2/2

== system TEST_Datcom/Vehicle System Model/Vehicle/Aerodynamics/Aerodynamic Coefficients/Aileron ==
  note: Aerodynamics coefficients for aileron and rudder will be modeled at a later time when 6DOF model is developed.
  Bus : Inport
  Constant1 : Constant  Value=0
  Mux1 : Mux  Inputs=6
  Terminator : Terminator
  delCoeff : Outport  VectorParamsAs1DForOutWhenUnconnected=off
  wires:
  Mux1/1 -> delCoeff/1
  Constant1/1 -> Mux1/1, Mux1/2, Mux1/3, Mux1/4, Mux1/5, Mux1/6
  Bus/1 -> Terminator/1

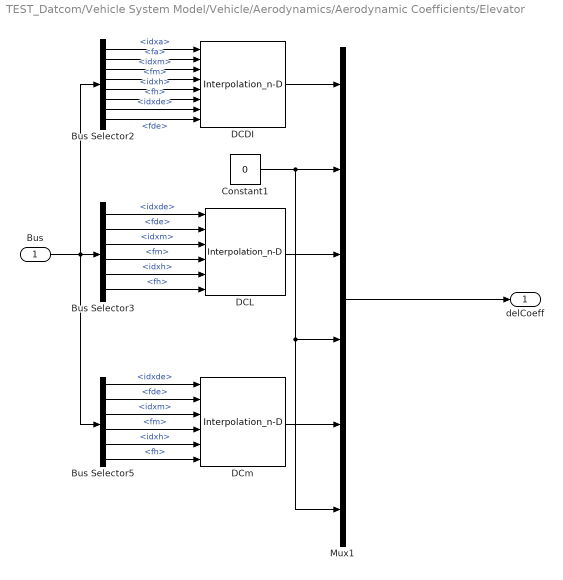
== system TEST_Datcom/Vehicle System Model/Vehicle/Aerodynamics/Aerodynamic Coefficients/Elevator ==
  Bus : Inport
  Bus Selector2 : BusSelector  OutputSignals=idxa,fa,idxm,fm,idxh,fh,idxde,fde
  Bus Selector3 : BusSelector  OutputSignals=idxde,fde,idxm,fm,idxh,fh
  Bus Selector5 : BusSelector  OutputSignals=idxde,fde,idxm,fm,idxh,fh
  Constant1 : Constant  Value=0
  DCDI : Interpolation_n-D  NumberOfTableDimensions=4  Table=permute(statdyn{1}.dcdi_sym,[1 3 4 2 ])  RemoveProtectionIndex=on
      settings: InputPortMap=u0,u1,u2,u3,u4,u5,u6,u7
  DCL : Interpolation_n-D  NumberOfTableDimensions=3  Table="permute(statdyn{1}.dcl_sym,[1  2  3])"  RemoveProtectionIndex=on
      settings: InputPortMap=u0,u1,u2,u3,u4,u5
  DCm : Interpolation_n-D  NumberOfTableDimensions=3  Table="permute(statdyn{1}.dcm_sym,[1  2  3])"  RemoveProtectionIndex=on
      settings: InputPortMap=u0,u1,u2,u3,u4,u5
  Mux1 : Mux  Inputs=6
  delCoeff : Outport  VectorParamsAs1DForOutWhenUnconnected=off
  wires:
  Mux1/1 -> delCoeff/1
  Bus/1 -> Bus Selector2/1, Bus Selector3/1, Bus Selector5/1
  DCDI/1 -> Mux1/1
  DCL/1 -> Mux1/3
  DCm/1 -> Mux1/5
  Constant1/1 -> Mux1/2, Mux1/4, Mux1/6
  Bus Selector2/1 -> DCDI/1  "<idxa>"
  Bus Selector2/2 -> DCDI/2  "<fa>"
  Bus Selector3/1 -> DCL/1  "<idxde>"
  Bus Selector3/2 -> DCL/2  "<fde>"
  Bus Selector5/1 -> DCm/1  "<idxde>"
  Bus Selector5/2 -> DCm/2  "<fde>"
  Bus Selector2/3 -> DCDI/3  "<idxm>"
  Bus Selector2/4 -> DCDI/4  "<fm>"
  Bus Selector2/5 -> DCDI/5  "<idxh>"
  Bus Selector2/6 -> DCDI/6  "<fh>"
  Bus Selector2/7 -> DCDI/7  "<idxde>"
  Bus Selector2/8 -> DCDI/8  "<fde>"
  Bus Selector3/3 -> DCL/3  "<idxm>"
  Bus Selector3/4 -> DCL/4  "<fm>"
  Bus Selector3/5 -> DCL/5  "<idxh>"
  Bus Selector3/6 -> DCL/6  "<fh>"
  Bus Selector5/3 -> DCm/3  "<idxm>"
  Bus Selector5/4 -> DCm/4  "<fm>"
  Bus Selector5/5 -> DCm/5  "<idxh>"
  Bus Selector5/6 -> DCm/6  "<fh>"

== system TEST_Datcom/Vehicle System Model/Vehicle/Aerodynamics/Aerodynamic Coefficients/Rudder ==
  note: Aerodynamics coefficients for aileron and rudder will be modeled at a later time when 6DOF model is developed.
  Bus : Inport
  Constant1 : Constant  Value=0
  Mux1 : Mux  Inputs=6
  Terminator : Terminator
  delCoeff : Outport  VectorParamsAs1DForOutWhenUnconnected=off
  wires:
  Mux1/1 -> delCoeff/1
  Constant1/1 -> Mux1/6, Mux1/5, Mux1/4, Mux1/3, Mux1/2, Mux1/1
  Bus/1 -> Terminator/1
